simulink model "hybrid_force_control"  (R2019a)
settings: Solver=VariableStepAuto  StartTime=0.0  StopTime=10.0  RelTol=1e-3
values from neighbouring files (symbols this model uses):
  wayPoints = [-0.7 -1.0 0.55;-0.5 -0.9 0.6;-0.3 -0.8 0.75;-0.1 -0.7 0.7;0.1 -0.6 0.75;0.3 -0.5 0.6;0.5 -0.45 0.65;0.7 -0.4 0.5]    [arm_traj.m]    (also in left_arm_tree.m = [0.6 0.6 0.2]; right_arm_tree.m = [0.6 -0.6 0.2])
undefined symbols (not defined in the file or in its folder): Sf, Sv, TsCtrl
libraries: dspinverses x6, robotmaniplib x5, simulink x2, vrlib x1, robotcorelib x1
settings Model: Creator=rajeshree  LastModifiedBy=rajeshree

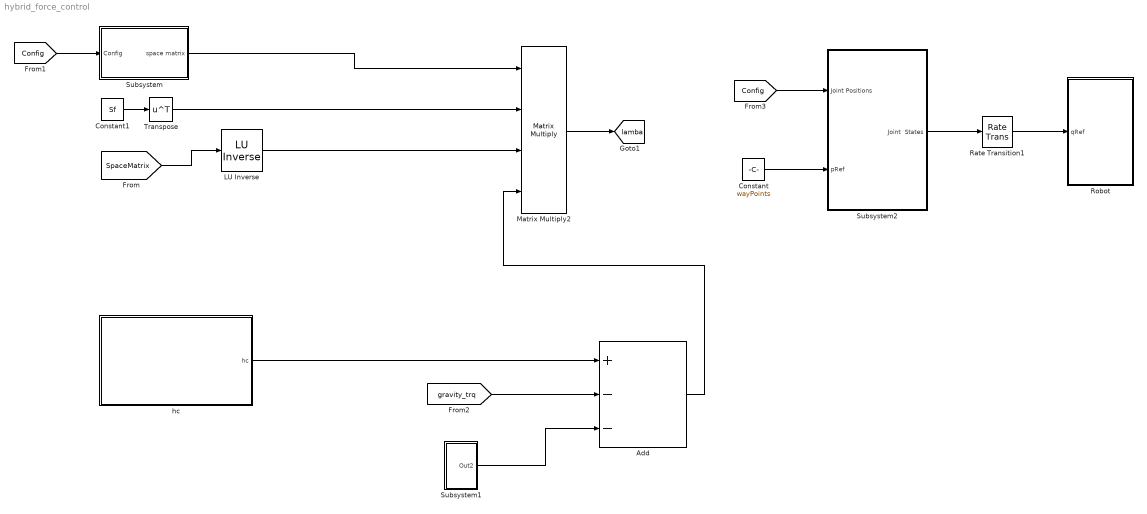
== system hybrid_force_control ==
  " LU Inverse" : dspinverses/ LU Inverse
      settings: SourceProductName=DSP System Toolbox
  Add : Sum  Inputs=+--
  Constant : Constant  Value=wayPoints
  Constant1 : Constant  Value=Sf
  Matrix Multiply2 : Product  Inputs=4  Multiplication=Matrix(*)
  Rate Transition1 : RateTransition  OutPortSampleTimeOpt=Inherit
  "Robot " : Subsystem
  Subsystem : Subsystem
  Subsystem1 : Subsystem
  Subsystem2 : Subsystem
  Transpose : Math  Operator=transpose  SaturateOnIntegerOverflow=on
  hc : Subsystem
  tag scope: lamba=global
  wires:
  Constant1/1 -> Transpose/1
  Subsystem/1(space matrix) -> Matrix Multiply2/1
  Transpose/1 -> Matrix Multiply2/2
  [SpaceMatrix] -> " LU Inverse"/1
  " LU Inverse"/1 -> Matrix Multiply2/3
  [Config] -> Subsystem/1(Config)
  Matrix Multiply2/1 -> [lamba]
  hc/1(hc) -> Add/1
  [gravity_trq] -> Add/2
  Add/1 -> Matrix Multiply2/4
  Subsystem1/1(Out2) -> Add/3
  Rate Transition1/1 -> "Robot "/1(qRef)
  Subsystem2/1(Joint  States) -> Rate Transition1/1
  [Config] -> Subsystem2/1(Joint Positions)
  Constant/1 -> Subsystem2/2(pRef)

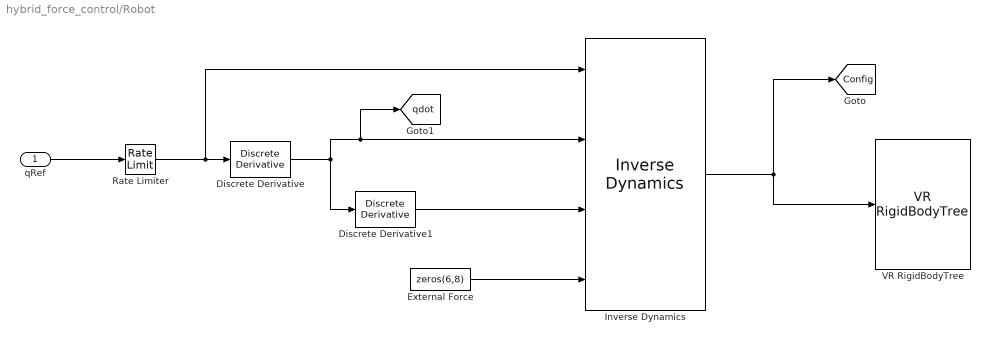
== system hybrid_force_control/Robot  ==
  qRef : Inport  SampleTime=TsCtrl
  Discrete Derivative : simulink/Discrete/Discrete Derivative  gainval=1.0  ICPrevScaledInput=0.0  OutMin=[]  OutMax=[]  OutDataType=fixdt(1, 16)  OutScaling=2^-10  DoSatur=off
  Discrete Derivative1 : simulink/Discrete/Discrete Derivative  gainval=1.0  ICPrevScaledInput=0.0  OutMin=[]  OutMax=[]  OutDataType=fixdt(1, 16)  OutScaling=2^-10  DoSatur=off
  External Force : Constant  Value=zeros(6,8)
  Inverse Dynamics : robotmaniplib/Inverse Dynamics  RigidBodyTree=newSubtree  SimulateUsing=Interpreted execution
      settings: SourceProductName=Robotics System Toolbox  SourceProductBaseCode=RO
  Rate Limiter : RateLimiter  RisingSlewLimit=pi  FallingSlewLimit=-pi  SampleTimeMode=inherited
  VR RigidBodyTree : vrlib/VR RigidBodyTree  RBT=newSubtree  useRBT=on  Ts=-1  ForceViewerOpen=on
      settings: SourceProductName=Simulink  SourceProductBaseCode=SL
  tag scope: Config=global, qdot=global
  wires:
  Discrete Derivative1/1 -> Inverse Dynamics/3
  Rate Limiter/1 -> Inverse Dynamics/1, Discrete Derivative/1
  Inverse Dynamics/1 -> VR RigidBodyTree/1, [Config]
  External Force/1 -> Inverse Dynamics/4
  Discrete Derivative/1 -> Discrete Derivative1/1, [qdot], Inverse Dynamics/2
  qRef/1 -> Rate Limiter/1

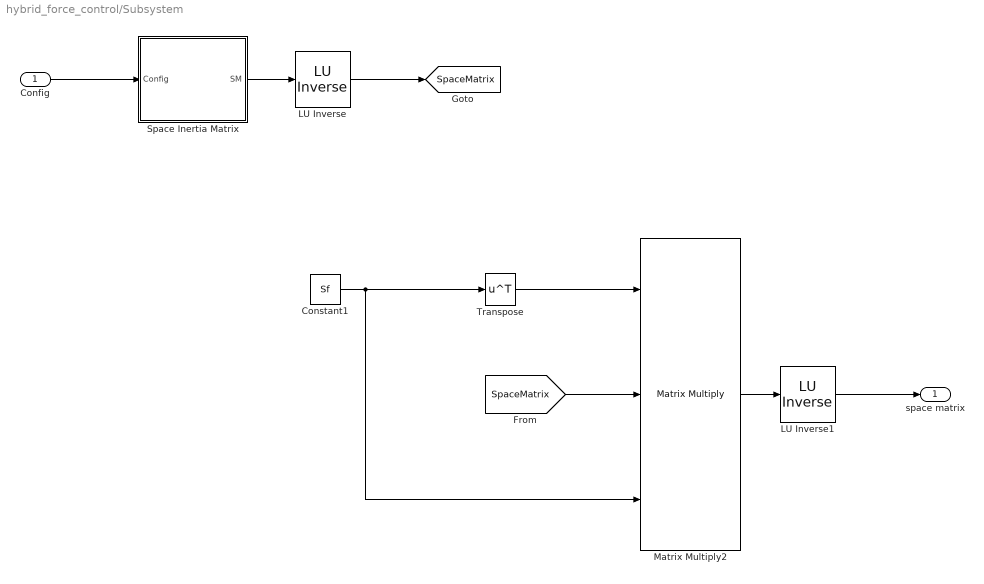
== system hybrid_force_control/Subsystem ==
  Config : Inport
  " LU Inverse" : dspinverses/ LU Inverse
      settings: SourceProductName=DSP System Toolbox
  " LU Inverse1" : dspinverses/ LU Inverse
      settings: SourceProductName=DSP System Toolbox
  Constant1 : Constant  Value=Sf
  Matrix Multiply2 : Product  Inputs=3  Multiplication=Matrix(*)
  Space Inertia Matrix : Subsystem
  Transpose : Math  Operator=transpose  SaturateOnIntegerOverflow=on
  space matrix : Outport
  tag scope: SpaceMatrix=global
  wires:
  " LU Inverse1"/1 -> space matrix/1
  Matrix Multiply2/1 -> " LU Inverse1"/1
  Transpose/1 -> Matrix Multiply2/1
  Space Inertia Matrix/1(SM) -> " LU Inverse"/1
  " LU Inverse"/1 -> [SpaceMatrix]
  Config/1 -> Space Inertia Matrix/1(Config)
  Constant1/1 -> Matrix Multiply2/3, Transpose/1
  [SpaceMatrix] -> Matrix Multiply2/2

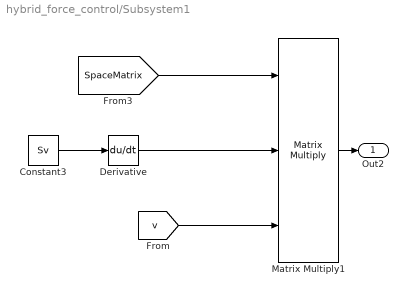
== system hybrid_force_control/Subsystem1 ==
  Constant3 : Constant  Value=Sv
  Derivative : Derivative
  Matrix Multiply1 : Product  Inputs=3  Multiplication=Matrix(*)
  Out2 : Outport
  wires:
  Matrix Multiply1/1 -> Out2/1
  Derivative/1 -> Matrix Multiply1/2
  [SpaceMatrix] -> Matrix Multiply1/1
  Constant3/1 -> Derivative/1
  [v] -> Matrix Multiply1/3

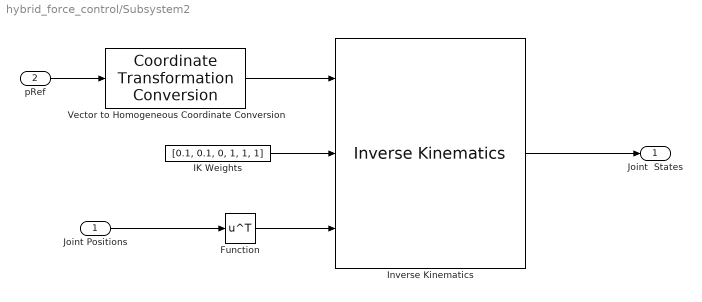
== system hybrid_force_control/Subsystem2 ==
  Joint Positions : Inport
  pRef : Inport  Port=2
  Function : Math  Operator=transpose  SaturateOnIntegerOverflow=on
  IK Weights : Constant  Value=[0.1, 0.1, 0, 1, 1, 1]
  Inverse Kinematics : robotmaniplib/Inverse Kinematics  RigidBodyTree=newSubtree  EndEffector=r_hand  ShowInfo=off  SolverName=BFGS Gradient Projection  EnforceJointLimits=on  MaxIterations=1500  MaxTime=10  GradientTolerance=1e-7  SolutionTolerance=1e-6  StepTolerance=1e-14  ErrorChangeTolerance=1e-12  UseErrorDamping=on  DampingBias=0.0025  SimulateUsing=Interpreted execution
      settings: SourceProductName=Robotics System Toolbox
  Vector to Homogeneous Coordinate Conversion : robotcorelib/Coordinate Transformation Conversion  InputRepresentation=Translation Vector  InputEulerSequence=ZYX  ShowTrVecInputPort=on  OutputRepresentation=Homogeneous Transformation  OutputEulerSequence=ZYX  ShowTrVecOutputPort=on  SimulateUsing=Interpreted execution
      settings: SourceProductBaseCode=RO
  Joint  States : Outport
  wires:
  Joint Positions/1 -> Function/1
  IK Weights/1 -> Inverse Kinematics/2
  pRef/1 -> Vector to Homogeneous Coordinate Conversion/1
  Function/1 -> Inverse Kinematics/3
  Vector to Homogeneous Coordinate Conversion/1 -> Inverse Kinematics/1
  Inverse Kinematics/1 -> Joint  States/1

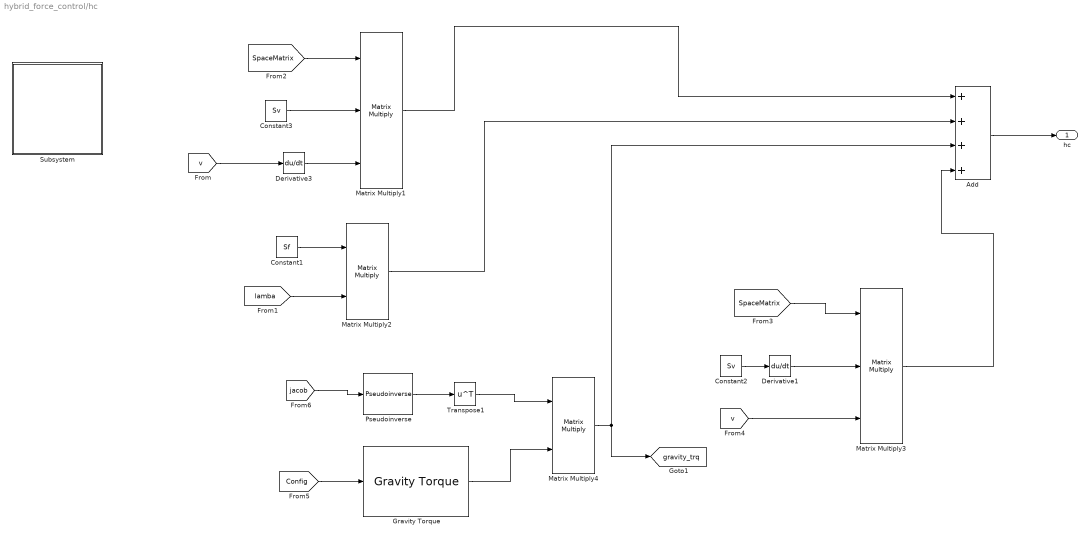
== system hybrid_force_control/hc ==
  Add : Sum  Inputs=++++
  Constant1 : Constant  Value=Sf
  Constant2 : Constant  Value=Sv
  Constant3 : Constant  Value=Sv
  Derivative1 : Derivative
  Derivative3 : Derivative
  Gravity Torque : robotmaniplib/Gravity Torque  RigidBodyTree=newSubtree  SimulateUsing=Interpreted execution
      settings: SourceProductName=Robotics System Toolbox
  Matrix Multiply1 : Product  Inputs=3  Multiplication=Matrix(*)
  Matrix Multiply2 : Product  Multiplication=Matrix(*)
  Matrix Multiply3 : Product  Inputs=3  Multiplication=Matrix(*)
  Matrix Multiply4 : Product  Multiplication=Matrix(*)
  Pseudoinverse : dspinverses/Pseudoinverse  wanterr=off  SimulateUsing=Interpreted execution
      settings: SourceProductName=DSP System Toolbox  SourceProductBaseCode=DS
  Subsystem : Subsystem
  Transpose1 : Math  Operator=transpose  SaturateOnIntegerOverflow=on
  hc : Outport
  tag scope: gravity_trq=global
  wires:
  Matrix Multiply1/1 -> Add/1
  [SpaceMatrix] -> Matrix Multiply1/1
  Constant1/1 -> Matrix Multiply2/1
  [lamba] -> Matrix Multiply2/2
  Matrix Multiply2/1 -> Add/2
  [Config] -> Gravity Torque/1
  Gravity Torque/1 -> Matrix Multiply4/2
  [jacob] -> Pseudoinverse/1
  Pseudoinverse/1 -> Transpose1/1
  Transpose1/1 -> Matrix Multiply4/1
  Matrix Multiply4/1 -> [gravity_trq], Add/3
  Add/1 -> hc/1
  Constant3/1 -> Matrix Multiply1/2
  Derivative3/1 -> Matrix Multiply1/3
  [SpaceMatrix] -> Matrix Multiply3/1
  Constant2/1 -> Derivative1/1
  Derivative1/1 -> Matrix Multiply3/2
  Matrix Multiply3/1 -> Add/4
  [v] -> Derivative3/1
  [v] -> Matrix Multiply3/3

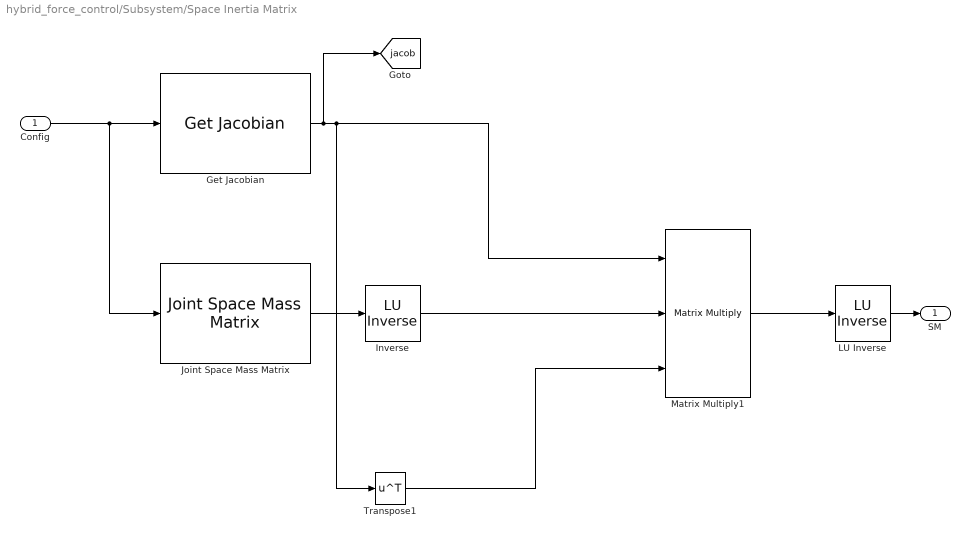
== system hybrid_force_control/Subsystem/Space Inertia Matrix ==
  Config : Inport
  " Inverse" : dspinverses/ LU Inverse
      settings: SourceProductName=DSP System Toolbox
  " LU Inverse" : dspinverses/ LU Inverse
      settings: SourceProductName=DSP System Toolbox
  Get Jacobian : robotmaniplib/Get Jacobian  RigidBodyTree=newSubtree  EndEffector=r_hand  SimulateUsing=Interpreted execution
      settings: SourceProductName=Robotics System Toolbox  SourceProductBaseCode=RO
  Joint Space Mass Matrix : robotmaniplib/Joint Space Mass Matrix  RigidBodyTree=newSubtree  SimulateUsing=Interpreted execution
      settings: SourceProductName=Robotics System Toolbox
  Matrix Multiply1 : Product  Inputs=3  Multiplication=Matrix(*)
  Transpose1 : Math  Operator=transpose  SaturateOnIntegerOverflow=on
  SM : Outport
  tag scope: jacob=global
  wires:
  Joint Space Mass Matrix/1 -> " Inverse"/1
  Transpose1/1 -> Matrix Multiply1/3
  Get Jacobian/1 -> [jacob], Transpose1/1, Matrix Multiply1/1
  " LU Inverse"/1 -> SM/1
  Config/1 -> Joint Space Mass Matrix/1, Get Jacobian/1
  Matrix Multiply1/1 -> " LU Inverse"/1
  " Inverse"/1 -> Matrix Multiply1/2

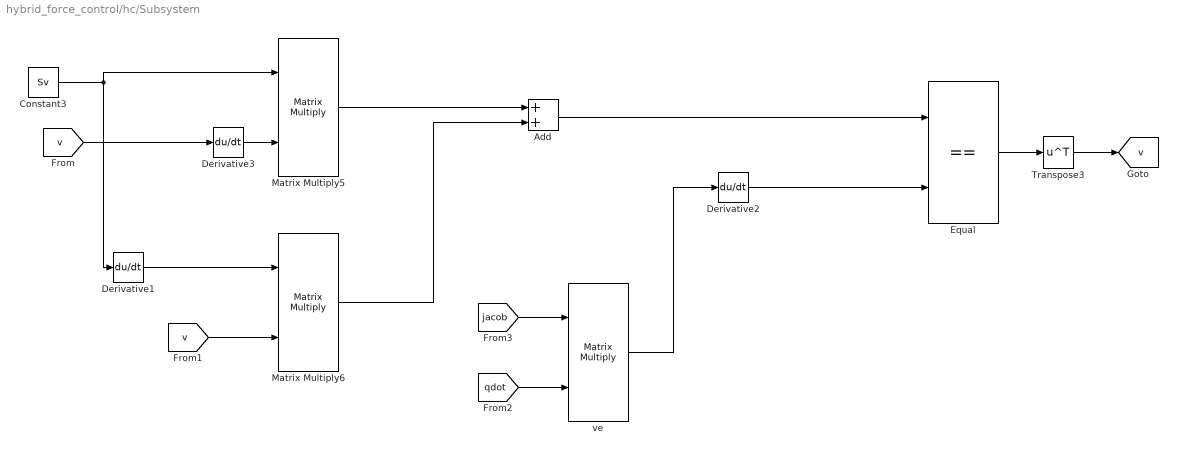
== system hybrid_force_control/hc/Subsystem ==
  Add : Sum
  Constant3 : Constant  Value=Sv
  Derivative1 : Derivative
  Derivative2 : Derivative
  Derivative3 : Derivative
  Equal : RelationalOperator  Operator===  OutDataTypeStr=boolean  RndMeth=Simplest
  Matrix Multiply5 : Product  Multiplication=Matrix(*)
  Matrix Multiply6 : Product  Multiplication=Matrix(*)
  Transpose3 : Math  Operator=transpose  SaturateOnIntegerOverflow=on
  ve : Product  Multiplication=Matrix(*)
  tag scope: v=global
  wires:
  Add/1 -> Equal/1
  Constant3/1 -> Derivative1/1, Matrix Multiply5/1
  Derivative1/1 -> Matrix Multiply6/1
  Derivative2/1 -> Equal/2
  Derivative3/1 -> Matrix Multiply5/2
  Matrix Multiply5/1 -> Add/1
  Matrix Multiply6/1 -> Add/2
  [qdot] -> ve/2
  [jacob] -> ve/1
  ve/1 -> Derivative2/1
  Equal/1 -> Transpose3/1
  [v] -> Derivative3/1
  Transpose3/1 -> [v]
  [v] -> Matrix Multiply6/2
